simulink model "wind_turbine"  (R2017b)
settings: Solver=VariableStepAuto  StartTime=0.0  StopTime=5  MaxStep=1e-4  RelTol=1e-3
libraries: powerlib x1
settings Model: Creator=el15kd  LastModifiedBy=el15kd

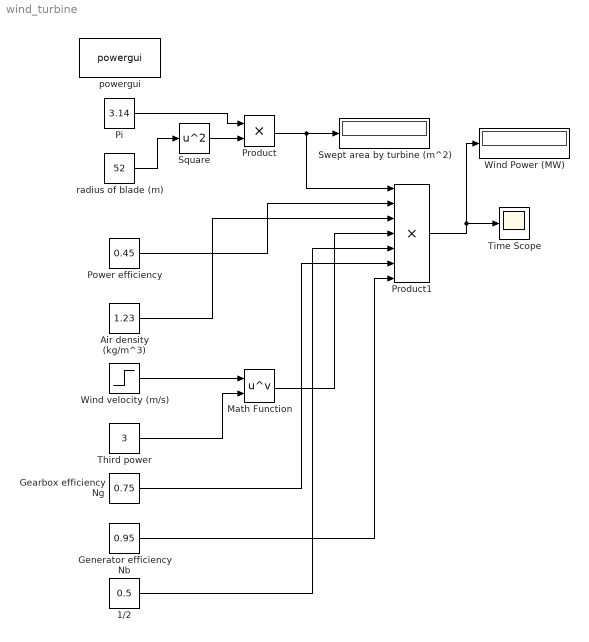
== system wind_turbine ==
  1/2 : Constant  Value=0.5
  Air density (kg/m^3) : Constant  Value=1.23
  Gearbox efficiency Ng : Constant  Value=0.75
  Generator efficiency Nb : Constant  Value=0.95
  Math Function : Math  Operator=pow  SaturateOnIntegerOverflow=on
  Pi : Constant  Value=3.14
  Power efficiency : Constant  Value=0.45
  Product : Product
  Product1 : Product  Inputs=7
  Square : Math  Operator=square  RndMeth=Zero  SaturateOnIntegerOverflow=on
  Swept area by turbine (m^2) : Display
  Third power : Constant  Value=3
  Time Scope : Scope
  Wind Power (MW) : Display
  Wind velocity (m/s) : Step  Before=1  After=30  SampleTime=0
  powergui : powerlib/powergui  Priority=1  SimulationMode=Continuous  SampleTime=50e-6  frequency=60  Iterations=50  frequencyindice=60  Pbase=100e6  ErrMax=1e-4  UnitsV=kV  UnitsW=MW  buscounter=0  FunctionMessages=off  echomessages=off  EnableUseOfTLC=off  CurrentSourceSwitches=off  DisableSnubberDevices=off  DisableRonSwitches=off  DisableVfSwitches=off  DisplayEquations=off  SolverType=Tustin/Backward Euler (TBE)  Interpol=off  ExternalGateDelay=off  methode=off  Ts=100  x0status=blocks  SPID=on  SwTol=0  HookPort=off  RestoreLinks=warning  ResistiveCurrentMeasurement=off  Frange=[0:2:500]  Ylog=off  Xlog=on  ShowGrid=off  save=off  variable=ZData  structure=0  ZoomFFT=off  StartTime=0.0  cycles=1  DisplayStyle=1  fundamental=60  FreqAxis=off  MaxFrequency=1000  frequencyindicesteady=1  RmsSteady=1  display=off
  radius of blade (m) : Constant  Value=52
  wires:
  radius of blade (m)/1 -> Square/1
  Square/1 -> Product/2
  Pi/1 -> Product/1
  Product/1 -> Product1/1, Swept area by turbine (m^2)/1
  Power efficiency/1 -> Product1/2
  Air density (kg/m^3)/1 -> Product1/3
  Third power/1 -> Math Function/2
  Wind velocity (m/s)/1 -> Math Function/1
  Math Function/1 -> Product1/4
  1/2/1 -> Product1/5
  Product1/1 -> Wind Power (MW)/1, Time Scope/1
  Gearbox efficiency Ng/1 -> Product1/6
  Generator efficiency Nb/1 -> Product1/7
